simulink model "TiltCopter_TOSTO_v4"  (R2015a)
settings: Solver=ode45  StartTime=0.0  StopTime=10  RelTol=1e-3
values from neighbouring files (symbols this model uses):
  A_Servo = [0 1 0; 0 0 1 ; -B0/B3 -B1/B3 -B2/B3]    [TiltCopter_Parameters_TOSTO_v3.m]
  b = 0.55/2    (= 0.275)    [TiltCopter_Parameters_TOSTO_v3.m]
  B_Servo = [0 ; 0 ; B0/B3]    [TiltCopter_Parameters_TOSTO_v3.m]
  C_Servo = eye(3)    [TiltCopter_Parameters_TOSTO_v3.m]
  degtorad = pi/180    (= 0.0174532925199)    [TiltCopter_Parameters_TOSTO_v3.m]
  dLMN = [dLdp  0    0 ... (first row only)    [TiltCopter_Parameters_TOSTO_v3.m]
  g = 9.81    [TiltCopter_Parameters_TOSTO_v3.m]
  I_Pi = diag([8.450e-5 8.450e-5 4.580e-5])    [TiltCopter_Parameters_TOSTO_v3.m]
  In = diag([Ixx Iyy Izz])    [TiltCopter_Parameters_TOSTO_v3.m]
  InInv = In\eye(3)    [TiltCopter_Parameters_TOSTO_v3.m]
  KaD = 5.4    [TiltCopter_Parameters_TOSTO_v3.m]
  KaI = 3.6    [TiltCopter_Parameters_TOSTO_v3.m]
  KaN = 38    [TiltCopter_Parameters_TOSTO_v3.m]
  KaP = 8.0    (= 8)    [TiltCopter_Parameters_TOSTO_v3.m]
  Kba = sqrt(KaD/KaI)    [TiltCopter_Parameters_TOSTO_v3.m]
  Kbp = sqrt(Kdp/Kip)    [TiltCopter_Parameters_TOSTO_v3.m]
  Kbq = sqrt(Kdq/Kiq)    [TiltCopter_Parameters_TOSTO_v3.m]
  Kbr = sqrt(Kdr/Kir)    [TiltCopter_Parameters_TOSTO_v3.m]
  Kdp = 0.0499    [TiltCopter_Parameters_TOSTO_v3.m]
  Kdq = 0.0499    [TiltCopter_Parameters_TOSTO_v3.m]
  Kdr = 0.0153    [TiltCopter_Parameters_TOSTO_v3.m]
  Kip = 0.304    [TiltCopter_Parameters_TOSTO_v3.m]
  Kiq = 0.304    [TiltCopter_Parameters_TOSTO_v3.m]
  Kir = 0.125    [TiltCopter_Parameters_TOSTO_v3.m]
  KPD = 0.00512    [TiltCopter_Parameters_TOSTO_v3.m]
  KPP = 1.61    [TiltCopter_Parameters_TOSTO_v3.m]
  Kpp = 0.298    [TiltCopter_Parameters_TOSTO_v3.m]
  Kpq = 0.298    [TiltCopter_Parameters_TOSTO_v3.m]
  Kpr = 0.135    [TiltCopter_Parameters_TOSTO_v3.m]
  Kq = Cq*ro*A*R^3    (= 2.88925724261e-07)    [TiltCopter_Parameters_TOSTO_v3.m]
  KRD = 0.00512    [TiltCopter_Parameters_TOSTO_v3.m]
  KRP = 1.61    [TiltCopter_Parameters_TOSTO_v3.m]
  Kt = Ct*ro*A*R^2    (= 2.46191978476e-05)    [TiltCopter_Parameters_TOSTO_v3.m]
  m = 1.510    (= 1.51)    [TiltCopter_Parameters_TOSTO_v3.m]
  m_servo = p(1)    [TiltCopter_Parameters_TOSTO_v3.m]
  Mb = diag([m m m])    [TiltCopter_Parameters_TOSTO_v3.m]
  MbInv = Mb\eye(3)    [TiltCopter_Parameters_TOSTO_v3.m]
  N = 1/Tf    (= 100)    [TiltCopter_Parameters_TOSTO_v3.m]
  omega_hover = OMEhov    [TiltCopter_Parameters_TOSTO_v3.m]
  pitchMax = pi/6    (= 0.523598775598)    [TiltCopter_Parameters_TOSTO_v3.m]
  q_servo = p(2)    [TiltCopter_Parameters_TOSTO_v3.m]
  rollMax = pi/6    (= 0.523598775598)    [TiltCopter_Parameters_TOSTO_v3.m]
  satp = 1.5    [TiltCopter_Parameters_TOSTO_v3.m]
  satq = 1.5    [TiltCopter_Parameters_TOSTO_v3.m]
  satr = 1    [TiltCopter_Parameters_TOSTO_v3.m]
  tau = 0.055257    [TiltCopter_Parameters_TOSTO_v3.m]
  U = [-1; 0; 0; 0]    [Main_tiltCopter_TOSTO_v3.m]
  x1 = [m q]    [TiltCopter_Parameters_TOSTO_v3.m]
  yawRateMax = pi/2    (= 1.57079632679)    [TiltCopter_Parameters_TOSTO_v3.m]
undefined symbols (not defined in the file or in its folder): KPI, KRI, sigbuilder_block
libraries: simulink x10, aerolibutil x10
(part 2 of 2)

== system TiltCopter_TOSTO_v4/TiltCopter/Actuators/External Momentum_2 ==
  tau_pi : Inport
  alpha_i : Inport  Port=2
  omega_i : Inport  Port=3
  motor_number : Inport  Port=4
  3x3 Cross Product : aerolibutil/3x3 Cross Product
  O_BPi : MATLAB Function  TreatAsAtomicUnit=on
  Product : Product  Multiplication=Matrix(*)
  Product1 : Product  Multiplication=Matrix(*)
  R_BP2 : MATLAB Function  TreatAsAtomicUnit=on
  Sum : Sum  Inputs=-+|
  Thrust computation : Subsystem
  M_i : Outport
  wires:
  Sum/1 -> M_i/1
  R_BP2/1(Rotation_matrix) -> Product1/1, Product/1
  alpha_i/1 -> R_BP2/1(alpha_2)
  Product/1 -> 3x3 Cross Product/2
  tau_pi/1 -> Product1/2
  motor_number/1 -> O_BPi/1(motor_number)
  omega_i/1 -> Thrust computation/1(omega_i)
  Thrust computation/1(Vector_Thrust_i) -> Product/2
  3x3 Cross Product/1 -> Sum/2
  Product1/1 -> Sum/1
  O_BPi/1(Origin_Rotation) -> 3x3 Cross Product/1

== system TiltCopter_TOSTO_v4/TiltCopter/Actuators/External Momentum_3 ==
  tau_pi : Inport
  alpha_i : Inport  Port=2
  omega_i : Inport  Port=3
  motor_number : Inport  Port=4
  3x3 Cross Product : aerolibutil/3x3 Cross Product
  O_BPi : MATLAB Function  TreatAsAtomicUnit=on
  Product : Product  Multiplication=Matrix(*)
  Product1 : Product  Multiplication=Matrix(*)
  R_BP3 : MATLAB Function  TreatAsAtomicUnit=on
  Sum : Sum  Inputs=-+|
  Thrust computation : Subsystem
  M_i : Outport
  wires:
  Sum/1 -> M_i/1
  R_BP3/1(Rotation_matrix) -> Product1/1, Product/1
  alpha_i/1 -> R_BP3/1(alpha_3)
  Product/1 -> 3x3 Cross Product/2
  tau_pi/1 -> Product1/2
  motor_number/1 -> O_BPi/1(motor_number)
  omega_i/1 -> Thrust computation/1(omega_i)
  Thrust computation/1(Vector_Thrust_i) -> Product/2
  3x3 Cross Product/1 -> Sum/2
  Product1/1 -> Sum/1
  O_BPi/1(Origin_Rotation) -> 3x3 Cross Product/1

== system TiltCopter_TOSTO_v4/TiltCopter/Actuators/External Momentum_4 ==
  tau_pi : Inport
  alpha_i : Inport  Port=2
  omega_i : Inport  Port=3
  motor_number : Inport  Port=4
  3x3 Cross Product : aerolibutil/3x3 Cross Product
  O_BPi : MATLAB Function  TreatAsAtomicUnit=on
  Product : Product  Multiplication=Matrix(*)
  Product1 : Product  Multiplication=Matrix(*)
  R_BP4 : MATLAB Function  TreatAsAtomicUnit=on
  Sum : Sum  Inputs=-+|
  Thrust computation : Subsystem
  M_i : Outport
  wires:
  Sum/1 -> M_i/1
  R_BP4/1(Rotation_matrix) -> Product1/1, Product/1
  alpha_i/1 -> R_BP4/1(alpha_4)
  Product/1 -> 3x3 Cross Product/2
  tau_pi/1 -> Product1/2
  motor_number/1 -> O_BPi/1(motor_number)
  omega_i/1 -> Thrust computation/1(omega_i)
  Thrust computation/1(Vector_Thrust_i) -> Product/2
  3x3 Cross Product/1 -> Sum/2
  Product1/1 -> Sum/1
  O_BPi/1(Origin_Rotation) -> 3x3 Cross Product/1

== system TiltCopter_TOSTO_v4/TiltCopter/Actuators/Servo_Motor 1 ==
  Pulse_1 [ms] : Inport
  "Angle [rad] -> Pulse [ms]" : Subsystem
  Demux : Demux  Outputs=3
  State-Space : StateSpace  A=A_Servo  B=B_Servo  C=C_Servo  D=[0 0 0]'  X0=[0 0 0 ]  ContinuousStateAttributes=['alpha' 'dalpha' 'ddalpha']
  alpha_1 [rad] : Outport
  dalpha_1 : Outport  Port=2
  ddalpha_1 : Outport  Port=3
  wires:
  "Angle [rad] -> Pulse [ms]"/1(Angle [rad]) -> State-Space/1
  Pulse_1 [ms]/1 -> "Angle [rad] -> Pulse [ms]"/1(Pulse [ms])
  State-Space/1 -> Demux/1
  Demux/1 -> alpha_1 [rad]/1
  Demux/2 -> dalpha_1/1
  Demux/3 -> ddalpha_1/1

== system TiltCopter_TOSTO_v4/TiltCopter/Actuators/Servo_Motor 2 ==
  Pulse_2 [ms] : Inport
  "Angle [rad] -> Pulse [ms]" : Subsystem
  Demux : Demux  Outputs=3
  State-Space : StateSpace  A=A_Servo  B=B_Servo  C=C_Servo  D=[0 0 0]'  X0=[0 0 0 ]  ContinuousStateAttributes=['alpha' 'dalpha' 'ddalpha']
  alpha_2 [rad] : Outport
  dalpha_2 : Outport  Port=2
  ddalpha_2 : Outport  Port=3
  wires:
  "Angle [rad] -> Pulse [ms]"/1(Angle [rad]) -> State-Space/1
  Pulse_2 [ms]/1 -> "Angle [rad] -> Pulse [ms]"/1(Pulse [ms])
  State-Space/1 -> Demux/1
  Demux/3 -> ddalpha_2/1
  Demux/2 -> dalpha_2/1
  Demux/1 -> alpha_2 [rad]/1

== system TiltCopter_TOSTO_v4/TiltCopter/Actuators/Servo_Motor 3 ==
  Pulse_3 [ms] : Inport
  "Angle [rad] -> Pulse [ms]" : Subsystem
  Demux : Demux  Outputs=3
  State-Space : StateSpace  A=A_Servo  B=B_Servo  C=C_Servo  D=[0 0 0]'  X0=[0 0 0 ]  ContinuousStateAttributes=['alpha' 'dalpha' 'ddalpha']
  alpha_3 [rad] : Outport
  dalpha_3 : Outport  Port=2
  ddalpha_3 : Outport  Port=3
  wires:
  "Angle [rad] -> Pulse [ms]"/1(Angle [rad]) -> State-Space/1
  Pulse_3 [ms]/1 -> "Angle [rad] -> Pulse [ms]"/1(Pulse [ms])
  State-Space/1 -> Demux/1
  Demux/1 -> alpha_3 [rad]/1
  Demux/2 -> dalpha_3/1
  Demux/3 -> ddalpha_3/1

== system TiltCopter_TOSTO_v4/TiltCopter/Actuators/Servo_Motor 4 ==
  Pulse_4 [ms] : Inport
  "Angle [rad] -> Pulse [ms]" : Subsystem
  Demux : Demux  Outputs=3
  State-Space : StateSpace  A=A_Servo  B=B_Servo  C=C_Servo  D=[0 0 0]'  X0=[0 0 0 ]  ContinuousStateAttributes=['alpha' 'dalpha' 'ddalpha']
  alpha_4 [rad] : Outport
  dalpha_4 : Outport  Port=2
  ddalpha_4 : Outport  Port=3
  wires:
  "Angle [rad] -> Pulse [ms]"/1(Angle [rad]) -> State-Space/1
  Pulse_4 [ms]/1 -> "Angle [rad] -> Pulse [ms]"/1(Pulse [ms])
  State-Space/1 -> Demux/1
  Demux/1 -> alpha_4 [rad]/1
  Demux/2 -> dalpha_4/1
  Demux/3 -> ddalpha_4/1

== system TiltCopter_TOSTO_v4/TiltCopter/Actuators/Traslational Force_1 ==
  alpha_i : Inport
  omega_i : Inport  Port=2
  Product : Product  Multiplication=Matrix(*)
  R_BP1 : MATLAB Function  TreatAsAtomicUnit=on
  Thrust computation : Subsystem
  F_i : Outport
  wires:
  Thrust computation/1(Vector_Thrust_i) -> Product/2
  Product/1 -> F_i/1
  omega_i/1 -> Thrust computation/1(omega_i)
  R_BP1/1(Rotation_matrix) -> Product/1
  alpha_i/1 -> R_BP1/1(alpha_1)

== system TiltCopter_TOSTO_v4/TiltCopter/Actuators/Traslational Force_2 ==
  alpha_i : Inport
  omega_i : Inport  Port=2
  Product : Product  Multiplication=Matrix(*)
  R_BP2 : MATLAB Function  TreatAsAtomicUnit=on
  Thrust computation : Subsystem
  F_i : Outport
  wires:
  Thrust computation/1(Vector_Thrust_i) -> Product/2
  Product/1 -> F_i/1
  omega_i/1 -> Thrust computation/1(omega_i)
  R_BP2/1(Rotation_matrix) -> Product/1
  alpha_i/1 -> R_BP2/1(alpha_2)

== system TiltCopter_TOSTO_v4/TiltCopter/Actuators/Traslational Force_3 ==
  alpha_i : Inport
  omega_i : Inport  Port=2
  Product : Product  Multiplication=Matrix(*)
  R_BP3 : MATLAB Function  TreatAsAtomicUnit=on
  Thrust computation : Subsystem
  F_i : Outport
  wires:
  Thrust computation/1(Vector_Thrust_i) -> Product/2
  Product/1 -> F_i/1
  omega_i/1 -> Thrust computation/1(omega_i)
  R_BP3/1(Rotation_matrix) -> Product/1
  alpha_i/1 -> R_BP3/1(alpha_3)

== system TiltCopter_TOSTO_v4/TiltCopter/Actuators/Traslational Force_4 ==
  alpha_i : Inport
  omega_i : Inport  Port=2
  Product : Product  Multiplication=Matrix(*)
  R_BP4 : MATLAB Function  TreatAsAtomicUnit=on
  Thrust computation : Subsystem
  F_i : Outport
  wires:
  Thrust computation/1(Vector_Thrust_i) -> Product/2
  Product/1 -> F_i/1
  omega_i/1 -> Thrust computation/1(omega_i)
  R_BP4/1(Rotation_matrix) -> Product/1
  alpha_i/1 -> R_BP4/1(alpha_4)

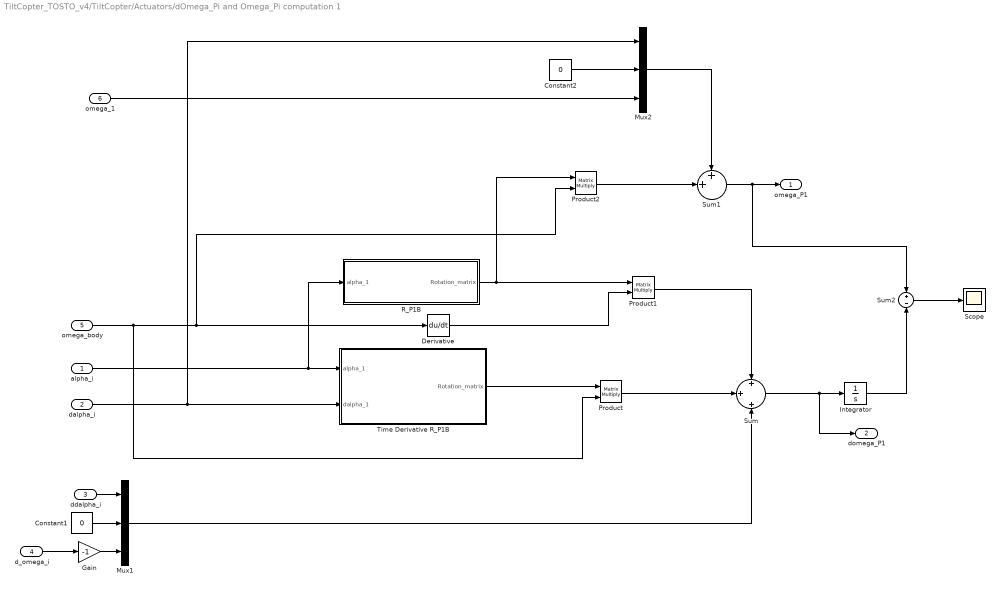
== system TiltCopter_TOSTO_v4/TiltCopter/Actuators/dOmega_Pi and Omega_Pi computation 1 ==
  alpha_i : Inport
  dalpha_i : Inport  Port=2
  ddalpha_i : Inport  Port=3
  d_omega_i : Inport  Port=4
  omega_body : Inport  Port=5
  omega_1 : Inport  Port=6
  Constant1 : Constant  Value=0
  Constant2 : Constant  Value=0
  Derivative : Derivative
  Gain : Gain  Gain=-1
  Integrator : Integrator
  Mux1 : Mux  Inputs=3
  Mux2 : Mux  Inputs=3
  Product : Product  Multiplication=Matrix(*)
  Product1 : Product  Multiplication=Matrix(*)
  Product2 : Product  Multiplication=Matrix(*)
  R_P1B : MATLAB Function  TreatAsAtomicUnit=on
  Scope : Scope
      settings: ShowLegends=on  SaveName=ScopeData29
  Sum : Sum  Inputs=+|+|+
  Sum1 : Sum  Inputs=++|
  Sum2 : Sum  Inputs=+-
  Time Derivative R_P1B : MATLAB Function  TreatAsAtomicUnit=on
  omega_P1 : Outport
  domega_P1 : Outport  Port=2
  wires:
  Derivative/1 -> Product1/2
  Product/1 -> Sum/2
  Time Derivative R_P1B/1(Rotation_matrix) -> Product/1
  Constant1/1 -> Mux1/2
  omega_body/1 -> Product/2, Product2/2, Derivative/1
  dalpha_i/1 -> Mux2/1, Time Derivative R_P1B/2(dalpha_1)
  alpha_i/1 -> R_P1B/1(alpha_1), Time Derivative R_P1B/1(alpha_1)
  R_P1B/1(Rotation_matrix) -> Product2/1, Product1/1
  Sum/1 -> domega_P1/1, Integrator/1
  Product1/1 -> Sum/1
  Mux1/1 -> Sum/3
  ddalpha_i/1 -> Mux1/1
  Product2/1 -> Sum1/2
  Constant2/1 -> Mux2/2
  Mux2/1 -> Sum1/1
  Sum1/1 -> Sum2/1, omega_P1/1
  omega_1/1 -> Mux2/3
  d_omega_i/1 -> Gain/1
  Integrator/1 -> Sum2/2
  Sum2/1 -> Scope/1
  Gain/1 -> Mux1/3

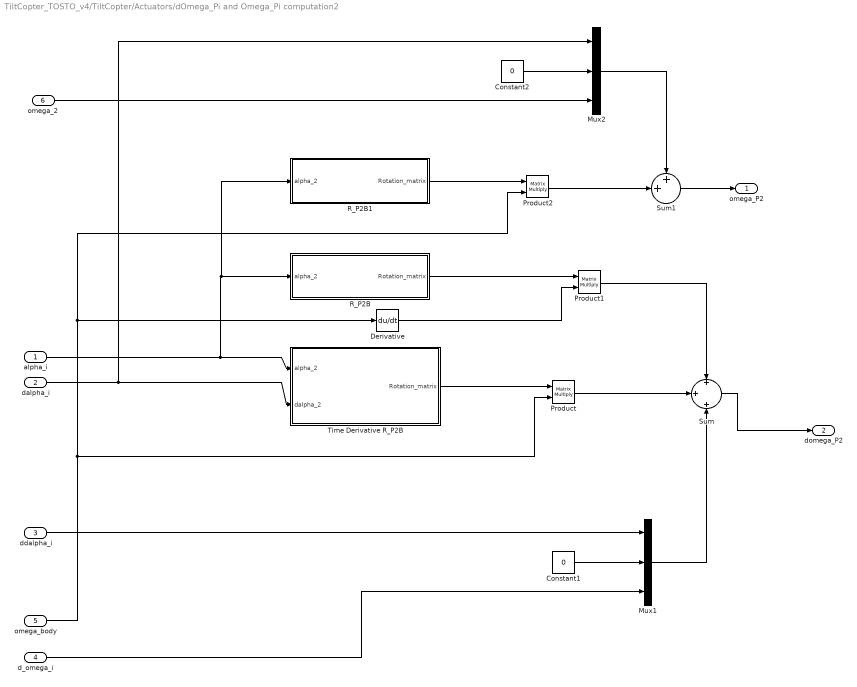
== system TiltCopter_TOSTO_v4/TiltCopter/Actuators/dOmega_Pi and Omega_Pi computation2 ==
  alpha_i : Inport
  dalpha_i : Inport  Port=2
  ddalpha_i : Inport  Port=3
  d_omega_i : Inport  Port=4
  omega_body : Inport  Port=5
  omega_2 : Inport  Port=6
  Constant1 : Constant  Value=0
  Constant2 : Constant  Value=0
  Derivative : Derivative
  Mux1 : Mux  Inputs=3
  Mux2 : Mux  Inputs=3
  Product : Product  Multiplication=Matrix(*)
  Product1 : Product  Multiplication=Matrix(*)
  Product2 : Product  Multiplication=Matrix(*)
  R_P2B : MATLAB Function  TreatAsAtomicUnit=on
  R_P2B1 : MATLAB Function  TreatAsAtomicUnit=on
  Sum : Sum  Inputs=+|+|+
  Sum1 : Sum  Inputs=++|
  Time Derivative R_P2B : MATLAB Function  TreatAsAtomicUnit=on
  omega_P2 : Outport
  domega_P2 : Outport  Port=2
  wires:
  Derivative/1 -> Product1/2
  Product/1 -> Sum/2
  Time Derivative R_P2B/1(Rotation_matrix) -> Product/1
  Constant1/1 -> Mux1/2
  omega_body/1 -> Product/2, Product2/2, Derivative/1
  dalpha_i/1 -> Mux2/1, Time Derivative R_P2B/2(dalpha_2)
  alpha_i/1 -> R_P2B1/1(alpha_2), R_P2B/1(alpha_2), Time Derivative R_P2B/1(alpha_2)
  Sum/1 -> domega_P2/1
  Product1/1 -> Sum/1
  Mux1/1 -> Sum/3
  ddalpha_i/1 -> Mux1/1
  R_P2B/1(Rotation_matrix) -> Product1/1
  R_P2B1/1(Rotation_matrix) -> Product2/1
  Product2/1 -> Sum1/2
  Constant2/1 -> Mux2/2
  Mux2/1 -> Sum1/1
  Sum1/1 -> omega_P2/1
  d_omega_i/1 -> Mux1/3
  omega_2/1 -> Mux2/3

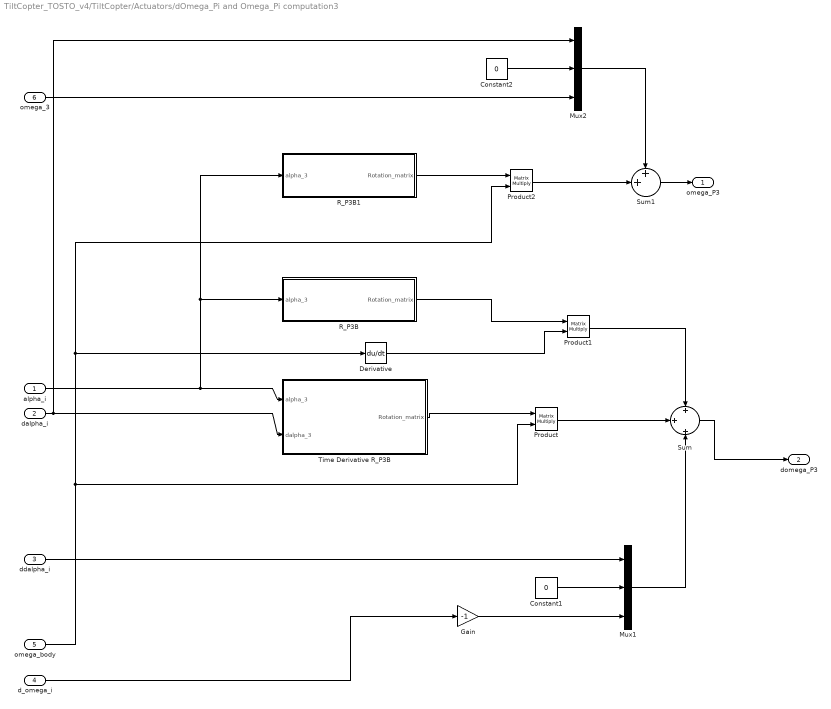
== system TiltCopter_TOSTO_v4/TiltCopter/Actuators/dOmega_Pi and Omega_Pi computation3 ==
  alpha_i : Inport
  dalpha_i : Inport  Port=2
  ddalpha_i : Inport  Port=3
  d_omega_i : Inport  Port=4
  omega_body : Inport  Port=5
  omega_3 : Inport  Port=6
  Constant1 : Constant  Value=0
  Constant2 : Constant  Value=0
  Derivative : Derivative
  Gain : Gain  Gain=-1
  Mux1 : Mux  Inputs=3
  Mux2 : Mux  Inputs=3
  Product : Product  Multiplication=Matrix(*)
  Product1 : Product  Multiplication=Matrix(*)
  Product2 : Product  Multiplication=Matrix(*)
  R_P3B : MATLAB Function  TreatAsAtomicUnit=on
  R_P3B1 : MATLAB Function  TreatAsAtomicUnit=on
  Sum : Sum  Inputs=+|+|+
  Sum1 : Sum  Inputs=++|
  Time Derivative R_P3B : MATLAB Function  TreatAsAtomicUnit=on
  omega_P3 : Outport
  domega_P3 : Outport  Port=2
  wires:
  Derivative/1 -> Product1/2
  Product/1 -> Sum/2
  Time Derivative R_P3B/1(Rotation_matrix) -> Product/1
  Constant1/1 -> Mux1/2
  omega_body/1 -> Product/2, Product2/2, Derivative/1
  alpha_i/1 -> R_P3B1/1(alpha_3), R_P3B/1(alpha_3), Time Derivative R_P3B/1(alpha_3)
  Sum/1 -> domega_P3/1
  Product1/1 -> Sum/1
  Mux1/1 -> Sum/3
  ddalpha_i/1 -> Mux1/1
  R_P3B/1(Rotation_matrix) -> Product1/1
  R_P3B1/1(Rotation_matrix) -> Product2/1
  Product2/1 -> Sum1/2
  Constant2/1 -> Mux2/2
  Mux2/1 -> Sum1/1
  dalpha_i/1 -> Mux2/1, Time Derivative R_P3B/2(dalpha_3)
  Sum1/1 -> omega_P3/1
  d_omega_i/1 -> Gain/1
  omega_3/1 -> Mux2/3
  Gain/1 -> Mux1/3

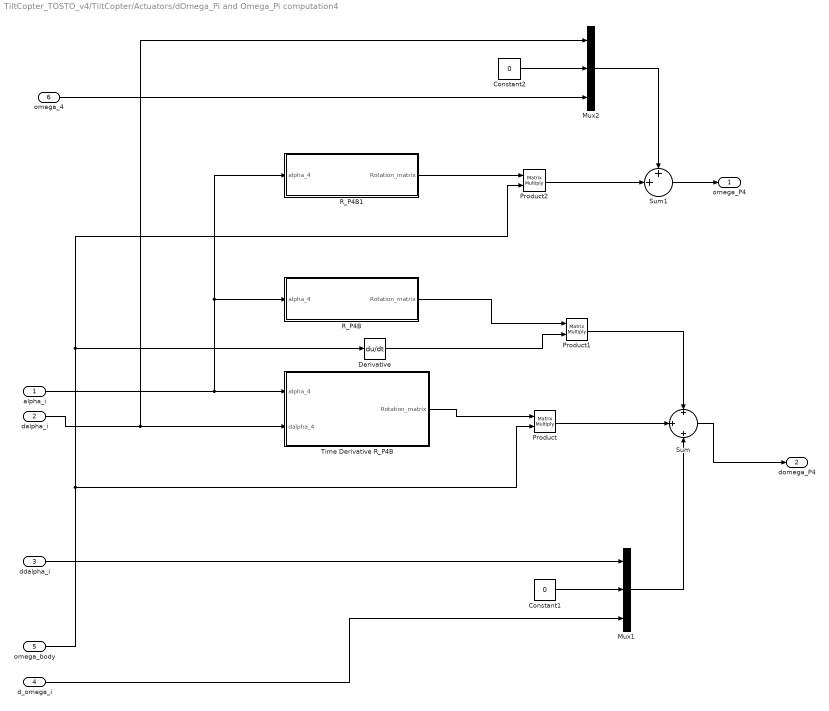
== system TiltCopter_TOSTO_v4/TiltCopter/Actuators/dOmega_Pi and Omega_Pi computation4 ==
  alpha_i : Inport
  dalpha_i : Inport  Port=2
  ddalpha_i : Inport  Port=3
  d_omega_i : Inport  Port=4
  omega_body : Inport  Port=5
  omega_4 : Inport  Port=6
  Constant1 : Constant  Value=0
  Constant2 : Constant  Value=0
  Derivative : Derivative
  Mux1 : Mux  Inputs=3
  Mux2 : Mux  Inputs=3
  Product : Product  Multiplication=Matrix(*)
  Product1 : Product  Multiplication=Matrix(*)
  Product2 : Product  Multiplication=Matrix(*)
  R_P4B : MATLAB Function  TreatAsAtomicUnit=on
  R_P4B1 : MATLAB Function  TreatAsAtomicUnit=on
  Sum : Sum  Inputs=+|+|+
  Sum1 : Sum  Inputs=++|
  Time Derivative R_P4B : MATLAB Function  TreatAsAtomicUnit=on
  omega_P4 : Outport
  domega_P4 : Outport  Port=2
  wires:
  Derivative/1 -> Product1/2
  Product/1 -> Sum/2
  Time Derivative R_P4B/1(Rotation_matrix) -> Product/1
  Constant1/1 -> Mux1/2
  omega_body/1 -> Product/2, Product2/2, Derivative/1
  dalpha_i/1 -> Mux2/1, Time Derivative R_P4B/2(dalpha_4)
  alpha_i/1 -> R_P4B1/1(alpha_4), R_P4B/1(alpha_4), Time Derivative R_P4B/1(alpha_4)
  Sum/1 -> domega_P4/1
  Product1/1 -> Sum/1
  Mux1/1 -> Sum/3
  ddalpha_i/1 -> Mux1/1
  R_P4B/1(Rotation_matrix) -> Product1/1
  Product2/1 -> Sum1/2
  Constant2/1 -> Mux2/2
  Mux2/1 -> Sum1/1
  R_P4B1/1(Rotation_matrix) -> Product2/1
  Sum1/1 -> omega_P4/1
  omega_4/1 -> Mux2/3
  d_omega_i/1 -> Mux1/3

== system TiltCopter_TOSTO_v4/TiltCopter/Actuators/tau_p1 computation ==
  omega_P1 : Inport
  domega_P1 : Inport  Port=2
  omega_i : Inport  Port=3
  3x3 Cross Product : aerolibutil/3x3 Cross Product
  Constant : Constant  Value=I_Pi
  Drag torque computation : Subsystem
  Gain : Gain  Gain=[1;1;-1]
  Product : Product  Multiplication=Matrix(*)
  Product1 : Product  Multiplication=Matrix(*)
  Sum : Sum  Inputs=+|+|-
  tau_P1 : Outport
  wires:
  Constant/1 -> Product/1, Product1/1
  omega_P1/1 -> 3x3 Cross Product/1, Product1/2
  Product/1 -> Sum/2
  domega_P1/1 -> Product/2
  Product1/1 -> 3x3 Cross Product/2
  Sum/1 -> tau_P1/1
  3x3 Cross Product/1 -> Sum/1
  Drag torque computation/1(Vector_DragTorque_i) -> Gain/1
  omega_i/1 -> Drag torque computation/1(omega_P1_z)
  Gain/1 -> Sum/3

== system TiltCopter_TOSTO_v4/TiltCopter/Actuators/tau_p2 computation ==
  omega_P2 : Inport
  domega_P2 : Inport  Port=2
  omega_i : Inport  Port=3
  3x3 Cross Product : aerolibutil/3x3 Cross Product
  Constant : Constant  Value=I_Pi
  Drag torque computation : Subsystem
  Gain : Gain  Gain=[1;1;-1]
  Product : Product  Multiplication=Matrix(*)
  Product1 : Product  Multiplication=Matrix(*)
  Sum : Sum  Inputs=+|+|-
  tau_P2 : Outport
  wires:
  3x3 Cross Product/1 -> Sum/1
  Sum/1 -> tau_P2/1
  Product1/1 -> 3x3 Cross Product/2
  domega_P2/1 -> Product/2
  Product/1 -> Sum/2
  omega_P2/1 -> Product1/2, 3x3 Cross Product/1
  Constant/1 -> Product/1, Product1/1
  Drag torque computation/1(Vector_DragTorque_i) -> Gain/1
  omega_i/1 -> Drag torque computation/1(omega_P2)
  Gain/1 -> Sum/3

== system TiltCopter_TOSTO_v4/TiltCopter/Actuators/tau_p3 computation1 ==
  omega_P3 : Inport
  domega_P3 : Inport  Port=2
  omega_i : Inport  Port=3
  3x3 Cross Product : aerolibutil/3x3 Cross Product
  Constant : Constant  Value=I_Pi
  Drag torque computation : Subsystem
  Gain : Gain  Gain=[1;1;-1]
  Product : Product  Multiplication=Matrix(*)
  Product1 : Product  Multiplication=Matrix(*)
  Sum : Sum  Inputs=+|+|-
  tau_P3 : Outport
  wires:
  Constant/1 -> Product1/1, Product/1
  omega_P3/1 -> 3x3 Cross Product/1, Product1/2
  Product/1 -> Sum/2
  domega_P3/1 -> Product/2
  Product1/1 -> 3x3 Cross Product/2
  Sum/1 -> tau_P3/1
  3x3 Cross Product/1 -> Sum/1
  Drag torque computation/1(Vector_DragTorque_i) -> Gain/1
  omega_i/1 -> Drag torque computation/1(omega_P3)
  Gain/1 -> Sum/3

== system TiltCopter_TOSTO_v4/TiltCopter/Actuators/tau_p4 computation2 ==
  omega_P4 : Inport
  domega_P4 : Inport  Port=2
  omega_i : Inport  Port=3
  3x3 Cross Product : aerolibutil/3x3 Cross Product
  Constant : Constant  Value=I_Pi
  Drag torque computation : Subsystem
  Gain : Gain  Gain=[1;1;-1]
  Product : Product  Multiplication=Matrix(*)
  Product1 : Product  Multiplication=Matrix(*)
  Sum : Sum  Inputs=+|+|-
  tau_P4 : Outport
  wires:
  3x3 Cross Product/1 -> Sum/1
  Sum/1 -> tau_P4/1
  Product1/1 -> 3x3 Cross Product/2
  domega_P4/1 -> Product/2
  Product/1 -> Sum/2
  omega_P4/1 -> Product1/2, 3x3 Cross Product/1
  Constant/1 -> Product/1, Product1/1
  Drag torque computation/1(Vector_DragTorque_i) -> Gain/1
  omega_i/1 -> Drag torque computation/1(omega_P4)
  Gain/1 -> Sum/3

== system TiltCopter_TOSTO_v4/TiltCopter/Actuators/ESC+Brushless1/Subsystem ==
  Throttle [%] : Inport
  Bias : Bias  Bias=x1(2)
  Gain : Gain  Gain=x1(1)
  Gain1 : Gain  Gain=-1/tau
  Gain2 : Gain  Gain=1/tau
  Gain3 : Gain  Gain=x1(1)
  Gain4 : Gain  Gain=x1(1)
  Sum : Sum  Inputs=|++
  Transfer Fcn : TransferFcn  Denominator=[(tau) 1]
  Transfer Fcn1 : TransferFcn  Denominator=[(tau) 1]
  omega_i : Outport
  domega_i : Outport  Port=2
  wires:
  Throttle [%]/1 -> Gain4/1, Transfer Fcn1/1, Transfer Fcn/1
  Transfer Fcn1/1 -> Gain1/1
  Gain1/1 -> Gain3/1
  Sum/1 -> domega_i/1
  Gain2/1 -> Sum/2
  Gain3/1 -> Sum/1
  Bias/1 -> omega_i/1
  Gain/1 -> Bias/1
  Transfer Fcn/1 -> Gain/1
  Gain4/1 -> Gain2/1

== system TiltCopter_TOSTO_v4/TiltCopter/Actuators/ESC+Brushless2/Subsystem ==
  Throttle [%] : Inport
  Bias : Bias  Bias=x1(2)
  Gain : Gain  Gain=x1(1)
  Gain1 : Gain  Gain=-1/tau
  Gain2 : Gain  Gain=1/tau
  Gain3 : Gain  Gain=x1(1)
  Gain4 : Gain  Gain=x1(1)
  Sum : Sum  Inputs=|++
  Transfer Fcn : TransferFcn  Denominator=[(tau) 1]
  Transfer Fcn1 : TransferFcn  Denominator=[(tau) 1]
  omega_i : Outport
  domega_i : Outport  Port=2
  wires:
  Throttle [%]/1 -> Gain4/1, Transfer Fcn1/1, Transfer Fcn/1
  Transfer Fcn1/1 -> Gain1/1
  Gain1/1 -> Gain3/1
  Sum/1 -> domega_i/1
  Gain2/1 -> Sum/2
  Gain3/1 -> Sum/1
  Bias/1 -> omega_i/1
  Gain/1 -> Bias/1
  Transfer Fcn/1 -> Gain/1
  Gain4/1 -> Gain2/1

== system TiltCopter_TOSTO_v4/TiltCopter/Actuators/ESC+Brushless3/Subsystem ==
  Throttle [%] : Inport
  Bias : Bias  Bias=x1(2)
  Gain : Gain  Gain=x1(1)
  Gain1 : Gain  Gain=-1/tau
  Gain2 : Gain  Gain=1/tau
  Gain3 : Gain  Gain=x1(1)
  Gain4 : Gain  Gain=x1(1)
  Sum : Sum  Inputs=|++
  Transfer Fcn : TransferFcn  Denominator=[(tau) 1]
  Transfer Fcn1 : TransferFcn  Denominator=[(tau) 1]
  omega_i : Outport
  domega_i : Outport  Port=2
  wires:
  Throttle [%]/1 -> Gain4/1, Transfer Fcn1/1, Transfer Fcn/1
  Transfer Fcn1/1 -> Gain1/1
  Gain1/1 -> Gain3/1
  Sum/1 -> domega_i/1
  Gain2/1 -> Sum/2
  Gain3/1 -> Sum/1
  Bias/1 -> omega_i/1
  Gain/1 -> Bias/1
  Transfer Fcn/1 -> Gain/1
  Gain4/1 -> Gain2/1

== system TiltCopter_TOSTO_v4/TiltCopter/Actuators/ESC+Brushless4/Subsystem ==
  Throttle [%] : Inport
  Bias : Bias  Bias=x1(2)
  Gain : Gain  Gain=x1(1)
  Gain1 : Gain  Gain=-1/tau
  Gain2 : Gain  Gain=1/tau
  Gain3 : Gain  Gain=x1(1)
  Gain4 : Gain  Gain=x1(1)
  Sum : Sum  Inputs=|++
  Transfer Fcn : TransferFcn  Denominator=[(tau) 1]
  Transfer Fcn1 : TransferFcn  Denominator=[(tau) 1]
  omega_i : Outport
  domega_i : Outport  Port=2
  wires:
  Throttle [%]/1 -> Gain4/1, Transfer Fcn1/1, Transfer Fcn/1
  Transfer Fcn1/1 -> Gain1/1
  Gain1/1 -> Gain3/1
  Sum/1 -> domega_i/1
  Gain2/1 -> Sum/2
  Gain3/1 -> Sum/1
  Bias/1 -> omega_i/1
  Gain/1 -> Bias/1
  Transfer Fcn/1 -> Gain/1
  Gain4/1 -> Gain2/1

== system TiltCopter_TOSTO_v4/TiltCopter/Actuators/External Momentum_1/Thrust computation ==
  omega_i : Inport
  Constant : Constant  Value=-Kt
  Constant1 : Constant  Value=0
  Constant2 : Constant  Value=0
  Mux : Mux  Inputs=3
  Product : Product
  Product1 : Product
  Vector_Thrust_i : Outport
  wires:
  Constant2/1 -> Mux/2
  omega_i/1 -> Product/2, Product/1
  Product/1 -> Product1/1
  Constant1/1 -> Mux/1
  Mux/1 -> Vector_Thrust_i/1
  Product1/1 -> Mux/3
  Constant/1 -> Product1/2

== system TiltCopter_TOSTO_v4/TiltCopter/Actuators/External Momentum_2/Thrust computation ==
  omega_i : Inport
  Constant : Constant  Value=-Kt
  Constant1 : Constant  Value=0
  Constant2 : Constant  Value=0
  Mux : Mux  Inputs=3
  Product : Product
  Product1 : Product
  Vector_Thrust_i : Outport
  wires:
  Constant2/1 -> Mux/2
  omega_i/1 -> Product/2, Product/1
  Product/1 -> Product1/1
  Constant1/1 -> Mux/1
  Mux/1 -> Vector_Thrust_i/1
  Product1/1 -> Mux/3
  Constant/1 -> Product1/2

== system TiltCopter_TOSTO_v4/TiltCopter/Actuators/External Momentum_3/Thrust computation ==
  omega_i : Inport
  Constant : Constant  Value=-Kt
  Constant1 : Constant  Value=0
  Constant2 : Constant  Value=0
  Mux : Mux  Inputs=3
  Product : Product
  Product1 : Product
  Vector_Thrust_i : Outport
  wires:
  Constant2/1 -> Mux/2
  omega_i/1 -> Product/2, Product/1
  Product/1 -> Product1/1
  Constant1/1 -> Mux/1
  Mux/1 -> Vector_Thrust_i/1
  Product1/1 -> Mux/3
  Constant/1 -> Product1/2

== system TiltCopter_TOSTO_v4/TiltCopter/Actuators/External Momentum_4/Thrust computation ==
  omega_i : Inport
  Constant : Constant  Value=-Kt
  Constant1 : Constant  Value=0
  Constant2 : Constant  Value=0
  Mux : Mux  Inputs=3
  Product : Product
  Product1 : Product
  Vector_Thrust_i : Outport
  wires:
  Constant2/1 -> Mux/2
  omega_i/1 -> Product/2, Product/1
  Product/1 -> Product1/1
  Constant1/1 -> Mux/1
  Mux/1 -> Vector_Thrust_i/1
  Product1/1 -> Mux/3
  Constant/1 -> Product1/2

== system TiltCopter_TOSTO_v4/TiltCopter/Actuators/Servo_Motor 1/Angle [rad] -> Pulse [ms] ==
  Pulse [ms] : Inport
  Add : Sum  Inputs=+-
  Constant : Constant  Value=q_servo
  Linear fitting gain : Gain  Gain=1/m_servo
  Angle [rad] : Outport
  wires:
  Constant/1 -> Add/2
  Add/1 -> Linear fitting gain/1
  Pulse [ms]/1 -> Add/1
  Linear fitting gain/1 -> Angle [rad]/1

== system TiltCopter_TOSTO_v4/TiltCopter/Actuators/Servo_Motor 2/Angle [rad] -> Pulse [ms] ==
  Pulse [ms] : Inport
  Add : Sum  Inputs=+-
  Constant : Constant  Value=q_servo
  Linear fitting gain : Gain  Gain=1/m_servo
  Angle [rad] : Outport
  wires:
  Constant/1 -> Add/2
  Add/1 -> Linear fitting gain/1
  Pulse [ms]/1 -> Add/1
  Linear fitting gain/1 -> Angle [rad]/1

== system TiltCopter_TOSTO_v4/TiltCopter/Actuators/Servo_Motor 3/Angle [rad] -> Pulse [ms] ==
  Pulse [ms] : Inport
  Add : Sum  Inputs=+-
  Constant : Constant  Value=q_servo
  Linear fitting gain : Gain  Gain=1/m_servo
  Angle [rad] : Outport
  wires:
  Constant/1 -> Add/2
  Add/1 -> Linear fitting gain/1
  Pulse [ms]/1 -> Add/1
  Linear fitting gain/1 -> Angle [rad]/1

== system TiltCopter_TOSTO_v4/TiltCopter/Actuators/Servo_Motor 4/Angle [rad] -> Pulse [ms] ==
  Pulse [ms] : Inport
  Add : Sum  Inputs=+-
  Constant : Constant  Value=q_servo
  Linear fitting gain : Gain  Gain=1/m_servo
  Angle [rad] : Outport
  wires:
  Constant/1 -> Add/2
  Add/1 -> Linear fitting gain/1
  Pulse [ms]/1 -> Add/1
  Linear fitting gain/1 -> Angle [rad]/1

== system TiltCopter_TOSTO_v4/TiltCopter/Actuators/Traslational Force_1/Thrust computation ==
  omega_i : Inport
  Constant : Constant  Value=-Kt
  Constant1 : Constant  Value=0
  Constant2 : Constant  Value=0
  Mux : Mux  Inputs=3
  Product : Product
  Product1 : Product
  Vector_Thrust_i : Outport
  wires:
  Constant2/1 -> Mux/2
  omega_i/1 -> Product/2, Product/1
  Product/1 -> Product1/1
  Constant1/1 -> Mux/1
  Mux/1 -> Vector_Thrust_i/1
  Product1/1 -> Mux/3
  Constant/1 -> Product1/2

== system TiltCopter_TOSTO_v4/TiltCopter/Actuators/Traslational Force_2/Thrust computation ==
  omega_i : Inport
  Constant : Constant  Value=-Kt
  Constant1 : Constant  Value=0
  Constant2 : Constant  Value=0
  Mux : Mux  Inputs=3
  Product : Product
  Product1 : Product
  Vector_Thrust_i : Outport
  wires:
  Constant2/1 -> Mux/2
  omega_i/1 -> Product/2, Product/1
  Product/1 -> Product1/1
  Constant1/1 -> Mux/1
  Mux/1 -> Vector_Thrust_i/1
  Product1/1 -> Mux/3
  Constant/1 -> Product1/2

== system TiltCopter_TOSTO_v4/TiltCopter/Actuators/Traslational Force_3/Thrust computation ==
  omega_i : Inport
  Constant : Constant  Value=-Kt
  Constant1 : Constant  Value=0
  Constant2 : Constant  Value=0
  Mux : Mux  Inputs=3
  Product : Product
  Product1 : Product
  Vector_Thrust_i : Outport
  wires:
  Constant2/1 -> Mux/2
  omega_i/1 -> Product/2, Product/1
  Product/1 -> Product1/1
  Constant1/1 -> Mux/1
  Mux/1 -> Vector_Thrust_i/1
  Product1/1 -> Mux/3
  Constant/1 -> Product1/2

== system TiltCopter_TOSTO_v4/TiltCopter/Actuators/Traslational Force_4/Thrust computation ==
  omega_i : Inport
  Constant : Constant  Value=-Kt
  Constant1 : Constant  Value=0
  Constant2 : Constant  Value=0
  Mux : Mux  Inputs=3
  Product : Product
  Product1 : Product
  Vector_Thrust_i : Outport
  wires:
  Constant2/1 -> Mux/2
  omega_i/1 -> Product/2, Product/1
  Product/1 -> Product1/1
  Constant1/1 -> Mux/1
  Mux/1 -> Vector_Thrust_i/1
  Product1/1 -> Mux/3
  Constant/1 -> Product1/2

== system TiltCopter_TOSTO_v4/TiltCopter/Actuators/tau_p1 computation/Drag torque computation ==
  omega_P1_z : Inport
  Constant : Constant  Value=-Kq
  Constant1 : Constant  Value=0
  Constant2 : Constant  Value=0
  Mux : Mux  Inputs=3
  Product : Product
  Product1 : Product
  Vector_DragTorque_i : Outport
  wires:
  Constant2/1 -> Mux/2
  Product/1 -> Product1/1
  Constant1/1 -> Mux/1
  Mux/1 -> Vector_DragTorque_i/1
  Product1/1 -> Mux/3
  Constant/1 -> Product1/2
  omega_P1_z/1 -> Product/2, Product/1

== system TiltCopter_TOSTO_v4/TiltCopter/Actuators/tau_p2 computation/Drag torque computation ==
  omega_P2 : Inport
  Constant : Constant  Value=Kq
  Constant1 : Constant  Value=0
  Constant2 : Constant  Value=0
  Mux : Mux  Inputs=3
  Product : Product
  Product1 : Product
  Vector_DragTorque_i : Outport
  wires:
  Constant2/1 -> Mux/2
  Product/1 -> Product1/1
  Constant1/1 -> Mux/1
  Mux/1 -> Vector_DragTorque_i/1
  Product1/1 -> Mux/3
  Constant/1 -> Product1/2
  omega_P2/1 -> Product/2, Product/1

== system TiltCopter_TOSTO_v4/TiltCopter/Actuators/tau_p3 computation1/Drag torque computation ==
  omega_P3 : Inport
  Constant : Constant  Value=-Kq
  Constant1 : Constant  Value=0
  Constant2 : Constant  Value=0
  Mux : Mux  Inputs=3
  Product : Product
  Product1 : Product
  Vector_DragTorque_i : Outport
  wires:
  Constant2/1 -> Mux/2
  Product/1 -> Product1/1
  Constant1/1 -> Mux/1
  Mux/1 -> Vector_DragTorque_i/1
  Product1/1 -> Mux/3
  Constant/1 -> Product1/2
  omega_P3/1 -> Product/2, Product/1

== system TiltCopter_TOSTO_v4/TiltCopter/Actuators/tau_p4 computation2/Drag torque computation ==
  omega_P4 : Inport
  Constant : Constant  Value=Kq
  Constant1 : Constant  Value=0
  Constant2 : Constant  Value=0
  Mux : Mux  Inputs=3
  Product : Product
  Product1 : Product
  Vector_DragTorque_i : Outport
  wires:
  Constant2/1 -> Mux/2
  Product/1 -> Product1/1
  Constant1/1 -> Mux/1
  Mux/1 -> Vector_DragTorque_i/1
  Product1/1 -> Mux/3
  Constant/1 -> Product1/2
  omega_P4/1 -> Product/2, Product/1

== matlab function TiltCopter_TOSTO_v4/TiltCopter/To body from Earth ==
  data: Alpha_e input; Earth input; body output
 function body = Tbe(Alpha_e, Earth)
%#codegen
phi = Alpha_e(1);
theta = Alpha_e(2);
psi = Alpha_e(3);

Sphi = sin(phi);
Cphi = cos(phi);
Stheta = sin(theta);
Ctheta = cos(theta);
Spsi = sin(psi);
Cpsi = cos(psi);

TBE = [        Ctheta*Cpsi               Ctheta*Spsi          -Stheta    ;
       Sphi*Stheta*Cpsi-Cphi*Spsi Sphi*Stheta*Spsi+Cphi*Cpsi Sphi*Ctheta ;
       Cphi*Stheta*Cpsi+Sphi*Spsi Cphi*Stheta*Spsi-Sphi*Cpsi Cphi*Ctheta];

body = TBE* Earth;

== matlab function TiltCopter_TOSTO_v4/TiltCopter/To Earth from body ==
  data: Alpha_e input; Earth output; body input
 function Earth = Tbet(Alpha_e, body)
%#codegen
phi = Alpha_e(1);
theta = Alpha_e(2);
psi = Alpha_e(3);

Sphi = sin(phi);
Cphi = cos(phi);
Stheta = sin(theta);
Ctheta = cos(theta);
Spsi = sin(psi);
Cpsi = cos(psi);

TBE = [        Ctheta*Cpsi               Ctheta*Spsi          -Stheta    ;
       Sphi*Stheta*Cpsi-Cphi*Spsi Sphi*Stheta*Spsi+Cphi*Cpsi Sphi*Ctheta ;
       Cphi*Stheta*Cpsi+Sphi*Spsi Cphi*Stheta*Spsi-Sphi*Cpsi Cphi*Ctheta];
TEB = TBE';

Earth = TEB* body;

== matlab function TiltCopter_TOSTO_v4/TiltCopter/To Earth from body_rates ==
  data: Alpha_e input; Rates_B input; Rates_E output
 function Rates_E = Einv(Alpha_e, Rates_B)
%#codegen
phi = Alpha_e(1);
theta = Alpha_e(2);

Sphi = sin(phi);
Cphi = cos(phi);
Ctheta = cos(theta);
Ttheta = tan(theta);

Einv = [1   Sphi*Ttheta    Cphi*Ttheta ;
        0       Cphi          -Sphi    ;
        0   Sphi/Ctheta    Cphi/Ctheta];

Rates_E = Einv* Rates_B;

== matlab function TiltCopter_TOSTO_v4/TiltCopter/Actuators/Traslational Force_1/R_BP1 ==
  data: Rotation_matrix output; alpha_1 input
function Rotation_matrix = fcn(alpha_1)
%#codegen

% Rotation matrix from group propeller 1 to body
R_BP1 = [ 1,0,0; 0, cos(alpha_1), -sin(alpha_1);0, sin(alpha_1),cos(alpha_1)];
      



Rotation_matrix = R_BP1;

== matlab function TiltCopter_TOSTO_v4/Mixer Function/NONLINEAR mixer/Inverted Linearized mixer matrix ==
  data: Fx input; Fy input; T input; L input; M input; N input; y output; omega_hover parameter; Kt parameter; Kq parameter; b parameter
function y = fcn(Fx,Fy,T,L,M,N,omega_hover,Kt,Kq,b)
%#codegen

omega_hover_sq = omega_hover^2;

% Linearized Mixer matrix (equilibrium points: omega = omega hover, alpha =
% 0

MM_param_jaco =[    0,     0,     0,    0,                   0,  -Kt*omega_hover_sq,                   0,   Kt*omega_hover_sq;
    0,     0,     0,    0,   Kt*omega_hover_sq,                   0,  -Kt*omega_hover_sq,                   0;
  -Kt,   -Kt,   -Kt,  -Kt,                   0,                   0,                   0,                   0;
    0, -Kt*b,     0, Kt*b,                   0,  -Kq*omega_hover_sq,                   0,   Kq*omega_hover_sq;
 Kt*b,     0, -Kt*b,    0,  -Kq*omega_hover_sq,                   0,   Kq*omega_hover_sq,                   0;
   Kq,   -Kq,    Kq,  -Kq, Kt*b*omega_hover_sq, Kt*b*omega_hover_sq, Kt*b*omega_hover_sq, Kt*b*omega_hover_sq];

% Compute the column vector result
W = [ eye(4)*0.001 zeros(4); zeros(4) eye(4)*10e8];
%W= eye(8);
result = wpinv(MM_param_jaco,W)*[Fx;Fy;T;L;M;N];
y = result;

== matlab function TiltCopter_TOSTO_v4/Controllers/Attitude Controller/To body from Earth_rates ==
  data: Alpha_e input; Rates_B output; Rates_E input
 function Rates_B = E(Alpha_e, Rates_E)
%#codegen
phi = Alpha_e(1);       % Roll
theta = Alpha_e(2);     % Pitch
psi = Alpha_e(3);       % Yaw

E = [cos(psi)*cos(theta),cos(theta)*sin(psi),-sin(theta);
 cos(psi)*sin(phi)*sin(theta) - cos(phi)*sin(psi), cos(phi)*cos(psi) + sin(phi)*sin(psi)*sin(theta), cos(theta)*sin(phi);
 sin(phi)*sin(psi) + cos(phi)*cos(psi)*sin(theta), cos(phi)*sin(psi)*sin(theta) - cos(psi)*sin(phi), cos(phi)*cos(theta)];

Rates_B = E* Rates_E;

== matlab function TiltCopter_TOSTO_v4/TiltCopter/Actuators/dOmega_Pi and Omega_Pi computation 1/Time Derivative R_P1B ==
  data: alpha_1 input; dalpha_1 input; Rotation_matrix output
function Rotation_matrix = fcn(alpha_1,dalpha_1)
%#codegen
dR_P1B = [ 0 0 0 ; 
          0 -sin(alpha_1) cos(alpha_1);
          0 -cos(alpha_1) -sin(alpha_1)];
      
Rotation_matrix = dR_P1B*dalpha_1;

== matlab function TiltCopter_TOSTO_v4/TiltCopter/Actuators/dOmega_Pi and Omega_Pi computation2/Time Derivative R_P2B ==
  data: alpha_2 input; dalpha_2 input; Rotation_matrix output
function Rotation_matrix = fcn(alpha_2,dalpha_2)
%#codegen
% omega_x = -dalpha_i;
% omega_y = 0;
% omega_z = 0;
% Define the skew simmetric matrix
% S = [0 -omega_z omega_y;omega_z 0 -omega_x; -omega_y omega_x 0];


%Time derivative of Rotation matrix from Body to propeller group 1
% This rotation matrix is obtained with the Skew symmetric matrix
% In fact R_dot = S(alpha) * R_BPi

dR_P2B = [ 0 0 0 ; sin(alpha_2) 0 cos(alpha_2);...
           cos(alpha_2) 0 -sin(alpha_2)];
      
Rotation_matrix = dR_P2B*dalpha_2;

== matlab function TiltCopter_TOSTO_v4/TiltCopter/Actuators/dOmega_Pi and Omega_Pi computation3/Time Derivative R_P3B ==
  data: alpha_3 input; dalpha_3 input; Rotation_matrix output
function Rotation_matrix = fcn(alpha_3,dalpha_3)
%#codegen
dR_P3B =[ 0 0 0 ; 0 sin(alpha_3) cos(alpha_3); 0 cos(alpha_3) -sin(alpha_3)]; 
      
Rotation_matrix = dR_P3B*dalpha_3;

== matlab function TiltCopter_TOSTO_v4/TiltCopter/Actuators/Traslational Force_2/R_BP2 ==
  data: Rotation_matrix output; alpha_2 input
function Rotation_matrix = fcn(alpha_2)
%#codegen

% Rotation matrix from Propeller group 2 to body
R_BP2 =[ 0, -cos(alpha_2), sin(alpha_2); 1,0,0; 0,sin(alpha_2),cos(alpha_2)];

Rotation_matrix =R_BP2;

== matlab function TiltCopter_TOSTO_v4/TiltCopter/Actuators/Traslational Force_3/R_BP3 ==
  data: Rotation_matrix output; alpha_3 input
function Rotation_matrix = fcn(alpha_3)
%#codegen

R_BP3 = [ -1, 0, 0;0, -cos(alpha_3), sin(alpha_3);0,  sin(alpha_3), cos(alpha_3)];

Rotation_matrix = R_BP3;

== matlab function TiltCopter_TOSTO_v4/TiltCopter/Actuators/Traslational Force_4/R_BP4 ==
  data: Rotation_matrix output; alpha_4 input
function Rotation_matrix = fcn(alpha_4)
%#codegen

R_BP4 = [0, cos(alpha_4), -sin(alpha_4); -1, 0, 0; 0, sin(alpha_4), cos(alpha_4)];

Rotation_matrix = R_BP4;

== matlab function TiltCopter_TOSTO_v4/TiltCopter/Actuators/dOmega_Pi and Omega_Pi computation4/Time Derivative R_P4B ==
  data: alpha_4 input; dalpha_4 input; Rotation_matrix output
function Rotation_matrix = fcn(alpha_4,dalpha_4)
%#codegen
dR_P4B = [ 0 0 0 ; -sin(alpha_4) 0 cos(alpha_4); -cos(alpha_4) 0 -sin(alpha_4)];
Rotation_matrix = dR_P4B*dalpha_4;

== matlab function TiltCopter_TOSTO_v4/TiltCopter/Actuators/External Momentum_1/O_BPi ==
  data: Origin_Rotation output; motor_number input; b parameter
function Origin_Rotation = fcn(motor_number,b)
%#codegen

% Rotation matrix from Body to propeller group
psi = (motor_number-1)*pi/2;


R_z = [cos(psi), -sin(psi), 0;
      sin(psi),  cos(psi), 0;
      0,         0, 1];
      



Origin_Rotation = R_z*[b;0;0];

== matlab function TiltCopter_TOSTO_v4/TiltCopter/Actuators/External Momentum_1/R_BP1 ==
  data: Rotation_matrix output; alpha_1 input
function Rotation_matrix = fcn(alpha_1)
%#codegen

% Rotation matrix from group propeller 1 to body
R_BP1 = [ 1,0,0; 0, cos(alpha_1), -sin(alpha_1);0, sin(alpha_1),cos(alpha_1)];
      



Rotation_matrix = R_BP1;

== matlab function TiltCopter_TOSTO_v4/TiltCopter/Actuators/External Momentum_2/O_BPi ==
  data: Origin_Rotation output; motor_number input; b parameter
function Origin_Rotation = fcn(motor_number,b)
%#codegen

% Rotation matrix from Body to propeller group
psi = (motor_number-1)*pi/2;


R_z =[ cos(psi), -sin(psi), 0;
      sin(psi),  cos(psi), 0;
      0,         0, 1];
      



Origin_Rotation = R_z*[b;0;0];

== matlab function TiltCopter_TOSTO_v4/TiltCopter/Actuators/External Momentum_2/R_BP2 ==
  data: Rotation_matrix output; alpha_2 input
function Rotation_matrix = fcn(alpha_2)
%#codegen

% Rotation matrix from Propeller group 2 to body
R_BP2 =[ 0, -cos(alpha_2), sin(alpha_2); 1,0,0; 0,sin(alpha_2),cos(alpha_2)];

Rotation_matrix =R_BP2;

== matlab function TiltCopter_TOSTO_v4/TiltCopter/Actuators/External Momentum_3/O_BPi ==
  data: Origin_Rotation output; motor_number input; b parameter
function Origin_Rotation = fcn(motor_number,b)
%#codegen

% Rotation matrix from Body to propeller group
psi = (motor_number-1)*pi/2;


R_z = [cos(psi), -sin(psi), 0;
      sin(psi),  cos(psi), 0;
      0,         0, 1];
      



Origin_Rotation = R_z*[b;0;0];

== matlab function TiltCopter_TOSTO_v4/TiltCopter/Actuators/External Momentum_3/R_BP3 ==
  data: Rotation_matrix output; alpha_3 input
function Rotation_matrix = fcn(alpha_3)
%#codegen

R_BP3 = [ -1, 0, 0;0, -cos(alpha_3), sin(alpha_3);0,  sin(alpha_3), cos(alpha_3)];

Rotation_matrix = R_BP3;

== matlab function TiltCopter_TOSTO_v4/TiltCopter/Actuators/External Momentum_4/O_BPi ==
  data: Origin_Rotation output; motor_number input; b parameter
function Origin_Rotation = fcn(motor_number,b)
%#codegen

% Rotation matrix from Body to propeller group
psi = (motor_number-1)*pi/2;


R_z = [cos(psi), -sin(psi), 0;
      sin(psi),  cos(psi), 0;
      0,         0, 1];
      



Origin_Rotation = R_z*[b;0;0];

== matlab function TiltCopter_TOSTO_v4/TiltCopter/Actuators/External Momentum_4/R_BP4 ==
  data: Rotation_matrix output; alpha_4 input
function Rotation_matrix = fcn(alpha_4)
%#codegen

R_BP4 = [0, cos(alpha_4), -sin(alpha_4); -1, 0, 0; 0, sin(alpha_4), cos(alpha_4)];

Rotation_matrix = R_BP4;

== matlab function TiltCopter_TOSTO_v4/TiltCopter/Actuators/dOmega_Pi and Omega_Pi computation2/R_P2B ==
  data: alpha_2 input; Rotation_matrix output
function Rotation_matrix = fcn(alpha_2)
%#codegen
R_P2B = [0 1 0; -cos(alpha_2) 0 sin(alpha_2);sin(alpha_2) 0 cos(alpha_2)];
      
Rotation_matrix = R_P2B;

== matlab function TiltCopter_TOSTO_v4/TiltCopter/Actuators/dOmega_Pi and Omega_Pi computation3/R_P3B ==
  data: alpha_3 input; Rotation_matrix output
function Rotation_matrix = fcn(alpha_3)
%#codegen
R_P3B = [ -1 0 0 ; 0 -cos(alpha_3) sin(alpha_3); 0 sin(alpha_3) cos(alpha_3)];
      
Rotation_matrix = R_P3B;

== matlab function TiltCopter_TOSTO_v4/TiltCopter/Actuators/dOmega_Pi and Omega_Pi computation 1/R_P1B ==
  data: alpha_1 input; Rotation_matrix output
function Rotation_matrix = fcn(alpha_1)
%#codegen
R_P1B = [ 1 0 0 ; 0 cos(alpha_1) sin(alpha_1); 0 -sin(alpha_1) cos(alpha_1)];
      
Rotation_matrix = R_P1B;

== matlab function TiltCopter_TOSTO_v4/TiltCopter/Actuators/dOmega_Pi and Omega_Pi computation4/R_P4B ==
  data: alpha_4 input; Rotation_matrix output
function Rotation_matrix = fcn(alpha_4)
%#codegen
R_P4B = [0 -1 0; cos(alpha_4) 0 sin(alpha_4); -sin(alpha_4) 0 cos(alpha_4)];
      
Rotation_matrix = R_P4B;

== matlab function TiltCopter_TOSTO_v4/TiltCopter/Actuators/dOmega_Pi and Omega_Pi computation2/R_P2B1 ==
  data: alpha_2 input; Rotation_matrix output
function Rotation_matrix = fcn(alpha_2)
%#codegen
R_P2B = [0 1 0; -cos(alpha_2) 0 sin(alpha_2);sin(alpha_2) 0 cos(alpha_2)];
      
Rotation_matrix = R_P2B;

== matlab function TiltCopter_TOSTO_v4/TiltCopter/Actuators/dOmega_Pi and Omega_Pi computation3/R_P3B1 ==
  data: alpha_3 input; Rotation_matrix output
function Rotation_matrix = fcn(alpha_3)
%#codegen
R_P3B = [ -1 0 0 ; 0 -cos(alpha_3) sin(alpha_3); 0 sin(alpha_3) cos(alpha_3)];
      
Rotation_matrix = R_P3B;

== matlab function TiltCopter_TOSTO_v4/TiltCopter/Actuators/dOmega_Pi and Omega_Pi computation4/R_P4B1 ==
  data: alpha_4 input; Rotation_matrix output
function Rotation_matrix = fcn(alpha_4)
%#codegen
R_P4B = [0 -1 0; cos(alpha_4) 0 sin(alpha_4); -sin(alpha_4) 0 cos(alpha_4)];
      
Rotation_matrix = R_P4B;
